simulink model "NavStateMachine"  (R2016b)
settings: Solver=FixedStepDiscrete  StartTime=0.0  StopTime=inf  FixedStep=0.01  RelTol=1e-3
undefined symbols (not defined in the file or in its folder): Chart, nav_statemachine_lib
settings Model: Creator=chenjianhui  LastModifiedBy=chenjianhui
settings OptimizationCC: MaxStackSize=64
settings DebuggingCC: ParameterTunabilityLossMsg=error
settings HardwareCC: ProdBitPerLong=64  ProdHWDeviceType=Intel->x86-64 (Linux 64)
settings RTWCC: SystemTargetFile=ert.tlc  HardwareBoard=Robot Operating System (ROS)  TLCOptions="-aInlineSetEventsForThisBaseRateFcn=TLC_FALSE -aSuppressMultiTaskScheduler=TLC_FALSE  -aRateBasedStepFcn=0"  TemplateMakefile=ert_default_tmf  Description=Embedded Coder  GenerateReport=on  Toolchain=Catkin  IncludeHyperlinkInReport=on  LaunchReport=on  TargetLang=C++  GenerateTraceInfo=on  GenerateTraceReport=on  GenerateTraceReportSl=on  GenerateTraceReportSf=on  GenerateTraceReportEml=on
settings CodeAppCC: ForceParamTrailComments=on  IgnoreCustomStorageClasses=off  OperatorAnnotations=on  SimulinkDataObjDesc=on  SFDataObjDesc=on  MATLABFcnDesc=on  InsertBlockDesc=on  MATLABSourceComments=on

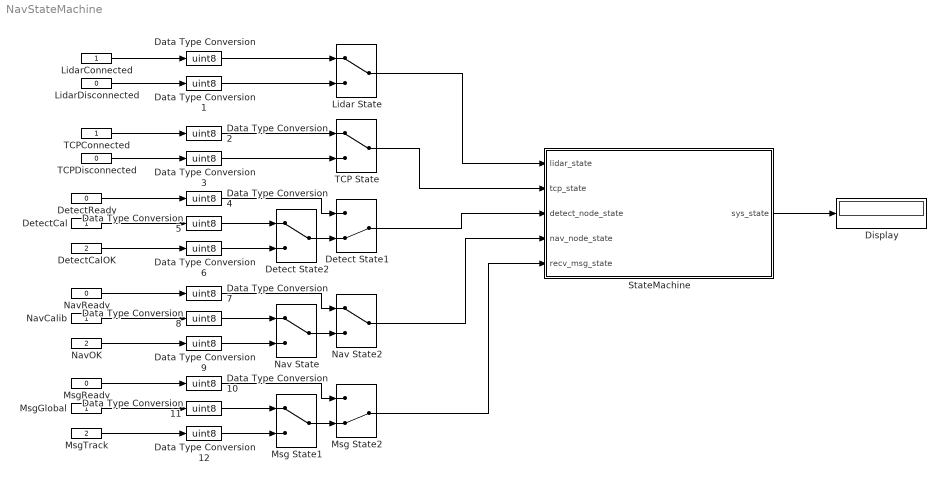
== system NavStateMachine ==
  Data Type Conversion{,1..12} (13 alike) : DataTypeConversion  OutDataTypeStr=uint8
  Detect State1 : ManualSwitch  CurrentSetting=0
  Detect State2 : ManualSwitch
  DetectCal : Constant
  DetectCalOK : Constant  Value=2
  DetectReady : Constant  Value=0
  Display : Display
  Lidar State : ManualSwitch
  LidarConnected : Constant
  LidarDisconnected : Constant  Value=0
  Msg State1 : ManualSwitch
  Msg State2 : ManualSwitch  CurrentSetting=0
  MsgGlobal : Constant
  MsgReady : Constant  Value=0
  MsgTrack : Constant  Value=2
  Nav State : ManualSwitch
  Nav State2 : ManualSwitch
  NavCalib : Constant
  NavOK : Constant  Value=2
  NavReady : Constant  Value=0
  StateMachine : Stateflow chart  AncestorBlock=nav_statemachine_lib/Chart  TreatAsAtomicUnit=on
  TCP State : ManualSwitch
  TCPConnected : Constant
  TCPDisconnected : Constant  Value=0
  wires:
  LidarConnected/1 -> Data Type Conversion/1
  LidarDisconnected/1 -> Data Type Conversion1/1
  StateMachine/1(sys_state) -> Display/1
  TCPConnected/1 -> Data Type Conversion2/1
  TCPDisconnected/1 -> Data Type Conversion3/1
  Lidar State/1 -> StateMachine/1(lidar_state)
  TCP State/1 -> StateMachine/2(tcp_state)
  Detect State2/1 -> Detect State1/2
  DetectReady/1 -> Data Type Conversion4/1
  DetectCal/1 -> Data Type Conversion5/1
  DetectCalOK/1 -> Data Type Conversion6/1
  Nav State/1 -> Nav State2/2
  NavReady/1 -> Data Type Conversion7/1
  NavCalib/1 -> Data Type Conversion8/1
  NavOK/1 -> Data Type Conversion9/1
  Msg State1/1 -> Msg State2/2
  MsgReady/1 -> Data Type Conversion10/1
  MsgGlobal/1 -> Data Type Conversion11/1
  MsgTrack/1 -> Data Type Conversion12/1
  Detect State1/1 -> StateMachine/3(detect_node_state)
  Nav State2/1 -> StateMachine/4(nav_node_state)
  Msg State2/1 -> StateMachine/5(recv_msg_state)
  Data Type Conversion/1 -> Lidar State/1
  Data Type Conversion1/1 -> Lidar State/2
  Data Type Conversion2/1 -> TCP State/1
  Data Type Conversion3/1 -> TCP State/2
  Data Type Conversion4/1 -> Detect State1/1
  Data Type Conversion5/1 -> Detect State2/1
  Data Type Conversion6/1 -> Detect State2/2
  Data Type Conversion7/1 -> Nav State2/1
  Data Type Conversion8/1 -> Nav State/1
  Data Type Conversion9/1 -> Nav State/2
  Data Type Conversion10/1 -> Msg State2/1
  Data Type Conversion11/1 -> Msg State1/1
  Data Type Conversion12/1 -> Msg State1/2

== stateflow chart NavStateMachine/StateMachine ==
  settings: updateMethod=DISCRETE  sampleTime=0.01
  state Ready
    sys_state = 1;
  state Initialization
    sys_state = 0;
  state GlobalLocationOK
    sys_state = 3;
  state GlobalLocationOn
    sys_state = 2;
  state SimuLocation
    sys_state = 4;
  (default) -> Initialization
  Initialization -> Ready : [lidar_state == 1 && ...
      | tcp_state == 1 && ...
      | detect_node_state == 0 && ...
      | nav_node_state == 0 && ...
      | recv_msg_state == 0]
  Ready -> Initialization [order 1] : [lidar_state == 0 || ...
      | tcp_state == 0]
  SimuLocation -> Initialization [order 1] : [lidar_state == 0 || ...
      | tcp_state == 0]
  GlobalLocationOK -> Initialization [order 1] : [lidar_state == 0 || ...
      | tcp_state == 0]
  GlobalLocationOn -> Initialization [order 1] : [lidar_state == 0 || ...
      | tcp_state == 0]
  Ready -> GlobalLocationOn [order 2] : [detect_node_state == 0 && ...
      | nav_node_state == 0 && ...
      | recv_msg_state == 1]
  GlobalLocationOn -> GlobalLocationOK [order 2] : [detect_node_state == 2]
  SimuLocation -> GlobalLocationOn [order 2] : [recv_msg_state == 1]
  GlobalLocationOK -> SimuLocation [order 2] : [nav_node_state == 2 && ...
      | recv_msg_state == 2]
  data: lidar_state input uint8; tcp_state input uint8; detect_node_state input uint8; nav_node_state input uint8; recv_msg_state input uint8; sys_state output uint8
